simulink model "STanque02"  (R2013a)
settings: Solver=ode45  StartTime=0.0  StopTime=100  RelTol=1e-3
undefined symbols (not defined in the file or in its folder): sigbuilder_block
settings Model: Creator=Cristhian Ivan  LastModifiedBy=Cristhian Ivan

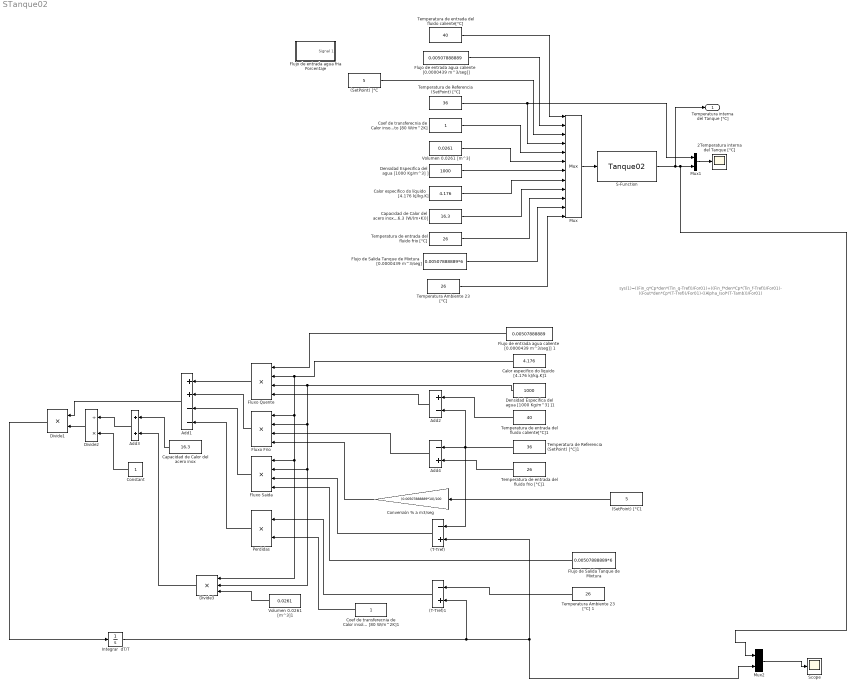
== system STanque02 ==
  note: sys(1)=((Fin_q*Cp*den*(Tin_q-Tref))/For01)+((Fin_f*den*Cp*(Tin_f-Tref))/For01)- ((Fout*den*Cp*(T-Tref))/For01)-((Alpha_Isol*(T-Tamb))/For01)
  (SetPoint) [°C : Constant  Value=5
  (SetPoint) [°C1 : Constant  Value=5
  (T-Tref) : Sum  Inputs=-+
  (T-Tref)1 : Sum  Inputs=-+
  2Temperatura interna del Tanque [°C] : Scope
      settings: TimeRange=10  YMin=35.9952  YMax=36
  Add1 : Sum  Inputs=++--
  Add2 : Sum  Inputs=+-
  Add3 : Sum
  Add4 : Sum  Inputs=-+
  Calor especifico do líquido  [4.176 kJ/kg.K] : Constant  Value=4.176
  Calor especifico do líquido  [4.176 kJ/kg.K]1 : Constant  Value=4.176
  "Capacidad de Calor del acero inox " : Constant  Value=16.3
  Capacidad de Calor del acero inox [16.3 (W/(m•K))] : Constant  Value=16.3
  Coef de transferecnia de Calor insolamiento [80 W/m^2K] : Constant
  Coef de transferecnia de Calor insolamiento [80 W/m^2K]1 : Constant
  Constant : Constant
  Conversión % a m3/seg : Gain  Gain=(0.00507888889*10)/100
  Densidad Especifica del agua [1000 Kg/m^3] ] : Constant  Value=1000
  Densidad Especifica del agua [1000 Kg/m^3] ]1 : Constant  Value=1000
  Divide1 : Product  Inputs=**
  Divide2 : Product  Inputs=/*
  Divide3 : Product  Inputs=***
  "Flujo de Salida Tanque de Mixtura " : Constant  Value=0.00507888889*6
  Flujo de Salida Tanque de Mixtura  [0.0000439 m^3/seg] : Constant  Value=0.00507888889*6
  "Flujo de entrada agua caliente  [0.0000439 m^3/seg]] " : Constant  Value=0.00507888889
  Flujo de entrada agua caliente  [0.0000439 m^3/seg]] 1 : Constant  Value=0.00507888889
  Flujo de entrada agua fria Porcentaje : Subsystem  Tag=STV Subsys  LoadFcn=sigbuilder_block('load');  StartFcn=sigbuilder_block('start');  StopFcn=sigbuilder_block('stop');  ClipboardFcn=sigbuilder_block('clipboard');  mask(Sigbuilder block){}
      mask help: Simulink:masks:SigbuilderBlock_MD
      mask init:
      | if ~strcmp(get_param(bdroot(gcbh),'SimulationStatus'),'stopped') tuvar = sigbuilder_block('maskInit'); end
      settings: CopyFcn=sigbuilder_block('copy');  DeleteFcn=sigbuilder_block('delete');  ModelCloseFcn=sigbuilder_block('modelClose');  PreSaveFcn=sigbuilder_block('preSave');  PauseFcn=sigbuilder_block('pause');  ContinueFcn=sigbuilder_block('continue');  NameChangeFcn=sigbuilder_block('namechange');  OpenFcn=sigbuilder_block('open',[6 28.5 1012.5 484.5 ]);  CloseFcn=sigbuilder_block('close');
      mask Display: plot(0, 0, 100, 100,[2, 2, 32, 32, 2], [68, 8, 8, 68, 68],[32, 2], [38, 38], [32, 19, 2],[53, 60, 44], [32, 17, 17, 2],[16, 16, 31, 31]);txt = getActiveGroup(gcbh);text(2, 100, txt,'verticalAlignment', 'top');
  Fluxo Frio : Product  Inputs=****
  Fluxo Quente : Product  Inputs=****
  Fluxo Saida : Product  Inputs=****
  Integrar  dT/T : Integrator
  Mux : Mux  Inputs=12
  Mux1 : Mux  Inputs=2
  Mux2 : Mux  Inputs=2
  Perdidas : Product  Inputs=**
  S-Function : S-Function  FunctionName=Tanque02  EnableBusSupport=off
  Scope : Scope
      settings: YMin=58.165  YMax=58.225
  "Temperatura Ambiente 23 [°C] " : Constant  Value=26
  Temperatura Ambiente 23 [°C] 1 : Constant  Value=26
  Temperatura de Referencia (SetPoint) [°C] : Constant  Value=36
  Temperatura de Referencia (SetPoint) [°C]1 : Constant  Value=36
  Temperatura de entrada del fluido caliente[°C] : Constant  Value=40
  Temperatura de entrada del fluido caliente[°C]1 : Constant  Value=40
  Temperatura de entrada del fluido frio [°C] : Constant  Value=26
  Temperatura de entrada del fluido frio [°C]1 : Constant  Value=26
  Volumen 0.0261 [m^3] : Constant  Value=0.0261
  Volumen 0.0261 [m^3]1 : Constant  Value=0.0261
  Temperatura interna del Tanque [°C] : Outport
  wires:
  Volumen 0.0261 [m^3]/1 -> Mux/6
  Capacidad de Calor del acero inox [16.3 (W/(m•K))]/1 -> Mux/9
  Calor especifico do líquido  [4.176 kJ/kg.K]/1 -> Mux/8
  Coef de transferecnia de Calor insolamiento [80 W/m^2K]/1 -> Mux/5
  Mux/1 -> S-Function/1
  Densidad Especifica del agua [1000 Kg/m^3] ]/1 -> Mux/7
  Temperatura de entrada del fluido caliente[°C]/1 -> Mux/1
  "Flujo de entrada agua caliente  [0.0000439 m^3/seg]] "/1 -> Mux/2
  Temperatura de Referencia (SetPoint) [°C]/1 -> Mux1/1, Mux/4
  Temperatura de entrada del fluido frio [°C]/1 -> Mux/10
  Flujo de Salida Tanque de Mixtura  [0.0000439 m^3/seg]/1 -> Mux/11
  "Temperatura Ambiente 23 [°C] "/1 -> Mux/12
  Mux1/1 -> 2Temperatura interna del Tanque [°C]/1
  (SetPoint) [°C/1 -> Mux/3
  Add1/1 -> Divide1/1
  Fluxo Quente/1 -> Add1/1
  Temperatura de entrada del fluido caliente[°C]1/1 -> Add2/1
  Add2/1 -> Fluxo Quente/4
  Calor especifico do líquido  [4.176 kJ/kg.K]1/1 -> Divide3/1, Fluxo Saida/1, Fluxo Frio/1, Fluxo Quente/2
  Densidad Especifica del agua [1000 Kg/m^3] ]1/1 -> Divide3/2, Fluxo Saida/2, Fluxo Frio/2, Fluxo Quente/3
  "Capacidad de Calor del acero inox "/1 -> Add3/1
  Divide3/1 -> Add3/2
  Volumen 0.0261 [m^3]1/1 -> Divide3/3
  (SetPoint) [°C1/1 -> Conversión % a m3/seg/1
  Conversión % a m3/seg/1 -> Fluxo Frio/4
  Fluxo Frio/1 -> Add1/2
  Temperatura de Referencia (SetPoint) [°C]1/1 -> (T-Tref)/1, Add4/1, Add2/2
  Divide1/1 -> Integrar  dT/T/1
  Integrar  dT/T/1 -> (T-Tref)1/2, (T-Tref)/2, Mux2/2
  (T-Tref)/1 -> Fluxo Saida/3
  "Flujo de Salida Tanque de Mixtura "/1 -> Fluxo Saida/4
  Flujo de entrada agua caliente  [0.0000439 m^3/seg]] 1/1 -> Fluxo Quente/1
  Fluxo Saida/1 -> Add1/3
  Perdidas/1 -> Add1/4
  Coef de transferecnia de Calor insolamiento [80 W/m^2K]1/1 -> Perdidas/2
  Temperatura Ambiente 23 [°C] 1/1 -> (T-Tref)1/1
  (T-Tref)1/1 -> Perdidas/1
  Add4/1 -> Fluxo Frio/3
  Temperatura de entrada del fluido frio [°C]1/1 -> Add4/2
  Add3/1 -> Divide2/1
  Divide2/1 -> Divide1/2
  Constant/1 -> Divide2/2
  S-Function/1 -> Mux2/1, Mux1/2, Temperatura interna del Tanque [°C]/1
  Mux2/1 -> Scope/1

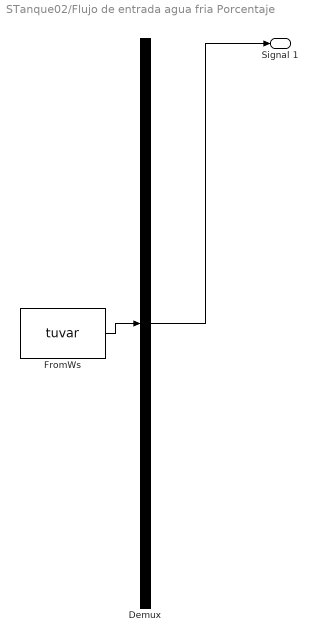
== system STanque02/Flujo de entrada agua fria Porcentaje ==
  Demux : Demux  Tag=STV Demux  Outputs=1
  FromWs : FromWorkspace  Tag=STV FromWs  VariableName=tuvar  SampleTime=0
      SigBuilderData=|
      | common.afterFinalStr = 'Extrapolate'
      | common.sampleTime = 0
      | dataSet.timeRange = [0 1000]
      | dataSet.name = 'Group 1'
      | sbobj.Groups.Name = 'Group 1'
      | sbobj.Groups.Signals.Name = 'Signal 1'
      | sbobj.Groups.Signals.XData = [0 2.8 2.8 200 200 401 401 600 600 800 800 1000]
      | sbobj.Groups.Signals.YData = [0 0 10 10 20 20 5 5 2.48e-05 2.48e-05 50 50]
      | sbobj.Groups.TimeRange = [0 1000]
  Signal 1 : Outport  Tag=STV Outport
  wires:
  Demux/1 -> Signal 1/1
  FromWs/1 -> Demux/1
